simulink model "c2837xd_ipc_cpu2_rx"  (R2021b)
settings: Solver=FixedStepDiscrete  StartTime=0.0  StopTime=inf  RelTol=1e-3  EnableMultiTasking=on
undefined symbols (not defined in the file or in its folder): C28x, CPU1, CPU2
libraries: c2837xDlib x4, c2000lib x1, demo_controls x1
settings Model: SimulationMode=external  ExtModeTrigDuration=8  Creator=The MathWorks, Inc.  LastModifiedBy=The MathWorks, Inc.
settings SolverCC: AlgebraicLoopSolver=TrustRegion  AutoInsertRateTranBlk=on  MinimalZcImpactIntegration=on
settings DataIOCC: ReturnWorkspaceOutputs=off
settings OptimizationCC: DefaultUnderspecifiedDataType=single  EnhancedBackFolding=on  StrengthReduction=on  PassReuseOutputArgsAs=Individual arguments  MaxStackSize=512  OptimizeBlockOrder=speed  DifferentSizesBufferReuse=on  EfficientTunableParamExpr=on
settings DebuggingCC: ParameterTunabilityLossMsg=error  SFMachineParentedDataDiag=warning  ArithmeticOperatorsInVariantConditions=warning
settings HardwareCC: ProdBitPerChar=16  ProdBitPerInt=16  ProdBitPerPointer=32  ProdBitPerSizeT=32  ProdBitPerPtrDiffT=32  ProdLargestAtomicInteger=Integer  ProdLargestAtomicFloat=None  ProdWordSize=16  ProdLongLongMode=on  ProdHWDeviceType=Texas Instruments->C2000
settings SFSimCC: SimUseLocalCustomCode=off  MATLABDynamicMemAlloc=off  CustomCodeUndefinedFunction=UseInterfaceOnly
settings RTWCC: Description=Embedded Coder  SystemTargetFile=ert.tlc  HardwareBoard=TI Delfino F2837xD  TemplateMakefile=ert_default_tmf  GenerateReport=on  RTWUseLocalCustomCode=off  Toolchain=Texas Instruments Code Composer Studio (C2000)  BuildConfiguration=Debug  IncludeHyperlinkInReport=on  LaunchReport=on  GenerateTraceInfo=on  GenerateTraceReport=on  GenerateTraceReportSl=on  GenerateTraceReportSf=on  GenerateTraceReportEml=on
settings CodeAppCC: ForceParamTrailComments=on  IgnoreCustomStorageClasses=off  OperatorAnnotations=on  SimulinkDataObjDesc=on  SFDataObjDesc=on  InsertBlockDesc=on
settings ERTTargetCC: CodeReplacementLibrary=TI C28x  ExtModeTransport=4  ExtModeStaticAlloc=on  ExtModeStaticAllocSize=10000  ExtModeMexFile=ext_xcp  ExtModeIntrfLevel=Level2 - Open

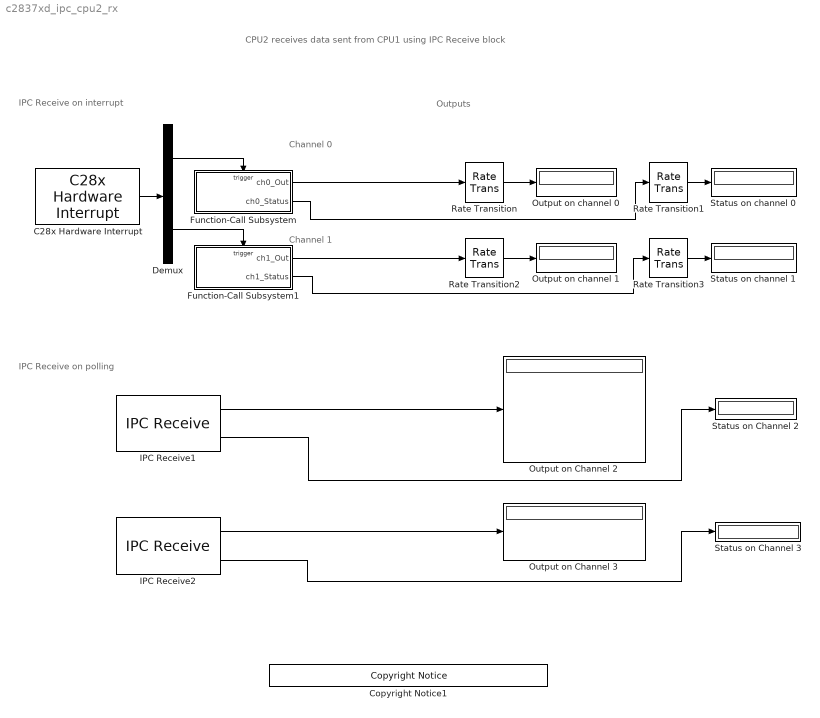
== system c2837xd_ipc_cpu2_rx ==
  note: Channel 0
  note: Channel 1
  note: IPC Receive on polling
  note: Outputs
  note: CPU2 receives data sent from CPU1
      | using IPC Receive block
  note: IPC Receive on interrupt
  C28x Hardware Interrupt : c2000lib/Scheduling/C28x Hardware Interrupt  irqnumbers=[1 1]  pienumbers=[13 14]  irqpriorities=[30 29]  irqpreempts=[1 1]  showinput=off  dspchiptype=C280X
      settings: SourceProductBaseCode=TIC2000
  Copyright Notice1 : demo_controls/Copyright Notice  year=2017  prod=tic2000
      settings: SourceProductBaseCode=ME
  Demux : Demux  Outputs=2
  Function-Call Subsystem : Subsystem  TreatAsAtomicUnit=on
  Function-Call Subsystem1 : Subsystem  TreatAsAtomicUnit=on
  IPC Receive1 : c2837xDlib/IPC Receive  blkParamProc=F2837x  SelectSource=C28x (CPU1/CPU2)  SelectChannel=2  DataType=uint16  DataLength=10  EnableBlocking=off  SampleTime=0.2
      settings: SourceProductBaseCode=TIC2000
  IPC Receive2 : c2837xDlib/IPC Receive  blkParamProc=F2837x  SelectSource=C28x (CPU1/CPU2)  SelectChannel=3  DataType=single  DataLength=3  EnableBlocking=off  SampleTime=.01
      settings: SourceProductBaseCode=TIC2000
  Output on Channel 2 : Display
  Output on Channel 3 : Display
  Output on channel 0 : Display
  Output on channel 1 : Display
  Rate Transition{,1..3} (4 alike) : RateTransition  Deterministic=off
  Status on Channel 2 : Display
  Status on Channel 3 : Display
  Status on channel 0 : Display
  Status on channel 1 : Display
  wires:
  IPC Receive2/1 -> Output on Channel 3/1
  IPC Receive1/1 -> Output on Channel 2/1
  IPC Receive1/2 -> Status on Channel 2/1
  IPC Receive2/2 -> Status on Channel 3/1
  Demux/2 -> Function-Call Subsystem1/Trigger
  C28x Hardware Interrupt/1 -> Demux/1
  Demux/1 -> Function-Call Subsystem/Trigger
  Function-Call Subsystem/1(ch0_Out) -> Rate Transition/1
  Function-Call Subsystem/2(ch0_Status) -> Rate Transition1/1
  Function-Call Subsystem1/1(ch1_Out) -> Rate Transition2/1
  Function-Call Subsystem1/2(ch1_Status) -> Rate Transition3/1
  Rate Transition/1 -> Output on channel 0/1
  Rate Transition1/1 -> Status on channel 0/1
  Rate Transition2/1 -> Output on channel 1/1
  Rate Transition3/1 -> Status on channel 1/1

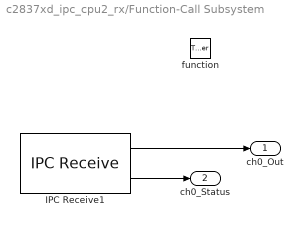
== system c2837xd_ipc_cpu2_rx/Function-Call Subsystem ==
  function : TriggerPort  TriggerType=function-call  VariantControl=Variant
  IPC Receive1 : c2837xDlib/IPC Receive  blkParamProc=F2837x  SelectSource=C28x (CPU1/CPU2)  SelectChannel=0  DataType=uint16  DataLength=1  EnableBlocking=off  SampleTime=-1
      settings: SourceProductBaseCode=TIC2000
  ch0_Out : Outport
  ch0_Status : Outport  Port=2
  wires:
  IPC Receive1/2 -> ch0_Status/1
  IPC Receive1/1 -> ch0_Out/1

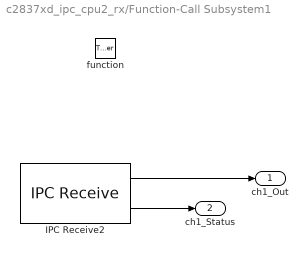
== system c2837xd_ipc_cpu2_rx/Function-Call Subsystem1 ==
  function : TriggerPort  TriggerType=function-call  VariantControl=Variant
  IPC Receive2 : c2837xDlib/IPC Receive  blkParamProc=F2837x  SelectSource=C28x (CPU1/CPU2)  SelectChannel=1  DataType=uint32  DataLength=1  EnableBlocking=off  SampleTime=-1
      settings: SourceProductBaseCode=TIC2000
  ch1_Out : Outport
  ch1_Status : Outport  Port=2
  wires:
  IPC Receive2/2 -> ch1_Status/1
  IPC Receive2/1 -> ch1_Out/1
